simulink model "Ejercicio1_modelo"  (R2020a)
settings: Solver=VariableStepAuto  StartTime=0.0  StopTime=5  RelTol=1e-3
values from neighbouring files (symbols this model uses):
  L = 500e-3    (= 0.5)    [Ejercicio1.m]    (also in Ejercicio5_parametros.m = 0.25)
  R = 100    [Ejercicio1.m]    (also in Ejercicio5_parametros.m = 0.5)
  v = 5    [Ejercicio1.m]
settings Model: Creator=juan  LastModifiedBy=juan

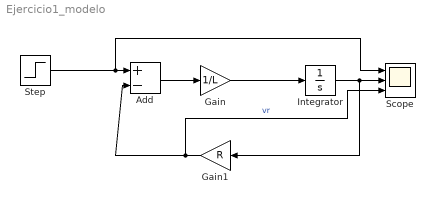
== system Ejercicio1_modelo ==
  Add : Sum  Inputs=+-
  Gain : Gain  Gain=1/L
  Gain1 : Gain  Gain=R
  Integrator : Integrator
  Scope : Scope  NumInputPorts=3
  Step : Step  After=v  SampleTime=0
  wires:
  Gain/1 -> Integrator/1
  Integrator/1 -> Gain1/1, Scope/2
  Add/1 -> Gain/1
  Gain1/1 -> Scope/3, Add/2  "vr"
  Step/1 -> Scope/1, Add/1
